simulink model "Cuantificador1"  (R2013a)
settings: Solver=ode45  StartTime=0.0  StopTime=1000  RelTol=1e-3
settings Model: Creator=Alfonso  LastModifiedBy=Alfonso

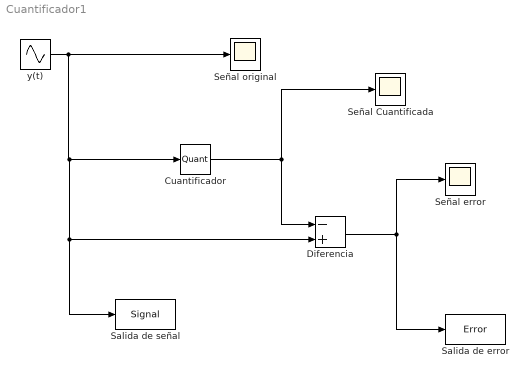
== system Cuantificador1 ==
  Cuantificador : Quantizer
  Diferencia : Sum  Inputs=-+
  Salida de error : ToWorkspace  VariableName=Error  SampleTime=-1
  Salida de señal : ToWorkspace  VariableName=Signal  SampleTime=-1
  Señal Cuantificada : Scope
  Señal error : Scope
      settings: SaveName=ScopeData2
  Señal original : Scope
  y(t) : Sin  SampleTime=0
  wires:
  y(t)/1 -> Salida de señal/1, Diferencia/2, Cuantificador/1, Señal original/1
  Cuantificador/1 -> Diferencia/1, Señal Cuantificada/1
  Diferencia/1 -> Señal error/1, Salida de error/1
